simulink model "D24P414_1_model02"  (R2021a)
settings: Solver=VariableStepAuto  StartTime=0.0  StopTime=7  FixedStep=1e-6  RelTol=1e-3
values from neighbouring files (symbols this model uses):
  p_ic = climate_p    [D24P414_1_script.m]
  params_fruit = fruit_p    [D24P414_1_script.m]
  t0_shift = days(t0-t0_12_00)    [D24P414_1_script.m]
  x0_fruit = fruit_ic    [D24P414_1_script.m]
  x0_ic = climate_ic    [D24P414_1_script.m]
libraries: HORTISIM x14
(part 2 of 2)

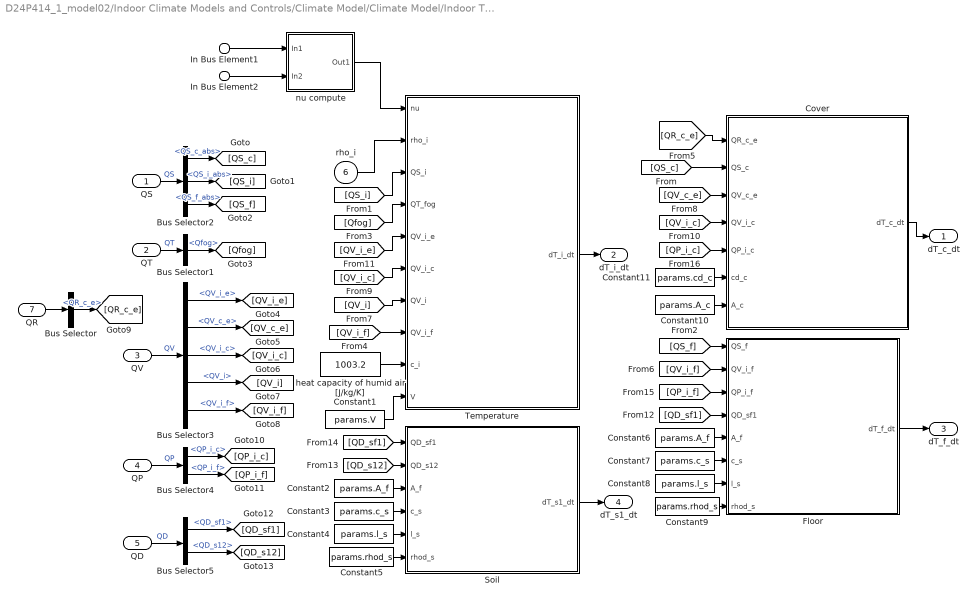
== system D24P414_1_model02/Indoor Climate Models and Controls/Climate Model/Climate Model/Indoor Temperature Model/Heat Balance ==
  QS : Inport
  QT : Inport  Port=2
  QV : Inport  Port=3
  QP : Inport  Port=4
  QD : Inport  Port=5
  rho_i : Inport  Port=6
  QR : Inport  Port=7
  In Bus Element1 : Inport  Port=8  PortName=screen  Element=beta
  In Bus Element2 : Inport  Port=8  PortName=screen  Element=value
  " Cover" : MATLAB Function  TreatAsAtomicUnit=on
  " Floor" : MATLAB Function  TreatAsAtomicUnit=on
  " Soil" : MATLAB Function  TreatAsAtomicUnit=on
  " Temperature" : MATLAB Function  TreatAsAtomicUnit=on
  Bus Selector : BusSelector  OutputSignals=QR_c_e
  Bus Selector1 : BusSelector  OutputSignals=Qfog
  Bus Selector2 : BusSelector  OutputSignals=QS_c_abs,QS_i_abs,QS_f_abs
  Bus Selector3 : BusSelector  OutputSignals=QV_i_e,QV_c_e,QV_i_c,QV_i,QV_i_f
  Bus Selector4 : BusSelector  OutputSignals=QP_i_c,QP_i_f
  Bus Selector5 : BusSelector  OutputSignals=QD_sf1,QD_s12
  Constant1 : Constant  Value=params.V
  Constant10 : Constant  Value=params.A_c
  Constant11 : Constant  Value=params.cd_c
  Constant2 : Constant  Value=params.A_f
  Constant3 : Constant  Value=params.c_s
  Constant4 : Constant  Value=params.l_s
  Constant5 : Constant  Value=params.rhod_s
  Constant6 : Constant  Value=params.A_f
  Constant7 : Constant  Value=params.c_s
  Constant8 : Constant  Value=params.l_s
  Constant9 : Constant  Value=params.rhod_s
  "heat capacity of humid air [J/kg/K] " : Constant  Value=1003.2
  nu compute : Subsystem
  dT_c_dt : Outport
  dT_i_dt : Outport  Port=2
  dT_f_dt : Outport  Port=3
  dT_s1_dt : Outport  Port=4
  wires:
  [QR_c_e] -> " Cover"/1(QR_c_e)
  Bus Selector/1 -> [QR_c_e]  "<QR_c_e>"
  QR/1 -> Bus Selector/1
  Constant11/1 -> " Cover"/6(cd_c)
  Constant10/1 -> " Cover"/7(A_c)
  Constant9/1 -> " Floor"/8(rhod_s)
  Constant8/1 -> " Floor"/7(l_s)
  Constant7/1 -> " Floor"/6(c_s)
  Constant6/1 -> " Floor"/5(A_f)
  Constant5/1 -> " Soil"/6(rhod_s)
  Constant4/1 -> " Soil"/5(l_s)
  Constant3/1 -> " Soil"/4(c_s)
  Constant2/1 -> " Soil"/3(A_f)
  Constant1/1 -> " Temperature"/10(V)
  "heat capacity of humid air [J/kg/K] "/1 -> " Temperature"/9(c_i)
  [QP_i_c] -> " Cover"/5(QP_i_c)
  [QP_i_f] -> " Floor"/3(QP_i_f)
  [QD_sf1] -> " Soil"/1(QD_sf1)
  [QD_s12] -> " Soil"/2(QD_s12)
  [QD_sf1] -> " Floor"/4(QD_sf1)
  Bus Selector5/2 -> [QD_s12]  "<QD_s12>"
  Bus Selector5/1 -> [QD_sf1]  "<QD_sf1>"
  Bus Selector4/2 -> [QP_i_f]  "<QP_i_f>"
  Bus Selector4/1 -> [QP_i_c]  "<QP_i_c>"
  [QV_i_e] -> " Temperature"/5(QV_i_e)
  [QV_i_c] -> " Cover"/4(QV_i_c)
  [QV_i_c] -> " Temperature"/6(QV_i_c)
  [QV_c_e] -> " Cover"/3(QV_c_e)
  [QV_i] -> " Temperature"/7(QV_i)
  [QV_i_f] -> " Floor"/2(QV_i_f)
  [QV_i_f] -> " Temperature"/8(QV_i_f)
  Bus Selector3/2 -> [QV_c_e]  "<QV_c_e>"
  Bus Selector3/3 -> [QV_i_c]  "<QV_i_c>"
  Bus Selector3/4 -> [QV_i]  "<QV_i>"
  Bus Selector3/5 -> [QV_i_f]  "<QV_i_f>"
  Bus Selector3/1 -> [QV_i_e]  "<QV_i_e>"
  [Qfog] -> " Temperature"/4(QT_fog)
  Bus Selector1/1 -> [Qfog]  "<Qfog>"
  [QS_f] -> " Floor"/1(QS_f)
  [QS_i] -> " Temperature"/3(QS_i)
  [QS_c] -> " Cover"/2(QS_c)
  Bus Selector2/3 -> [QS_f]  "<QS_f_abs>"
  Bus Selector2/2 -> [QS_i]  "<QS_i_abs>"
  Bus Selector2/1 -> [QS_c]  "<QS_c_abs>"
  " Cover"/1(dT_c_dt) -> dT_c_dt/1
  QV/1 -> Bus Selector3/1  "QV"
  rho_i/1 -> " Temperature"/2(rho_i)
  QP/1 -> Bus Selector4/1  "QP"
  QS/1 -> Bus Selector2/1  "QS"
  QT/1 -> Bus Selector1/1  "QT"
  " Temperature"/1(dT_i_dt) -> dT_i_dt/1
  QD/1 -> Bus Selector5/1  "QD"
  " Soil"/1(dT_s1_dt) -> dT_s1_dt/1
  " Floor"/1(dT_f_dt) -> dT_f_dt/1
  In Bus Element1/1 -> nu compute/1(In1)
  In Bus Element2/1 -> nu compute/2(In2)
  nu compute/1(Out1) -> " Temperature"/1(nu)

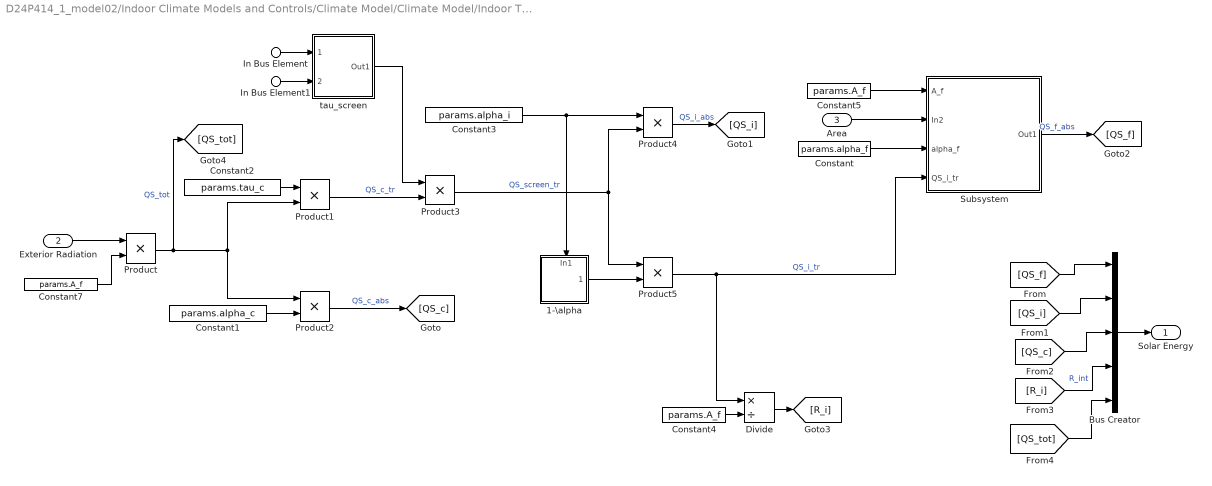
== system D24P414_1_model02/Indoor Climate Models and Controls/Climate Model/Climate Model/Indoor Temperature Model/Radiation Model ==
  In Bus Element : Inport  PortName=screen  Element=gamma_max
  In Bus Element1 : Inport  PortName=screen  Element=value
  Exterior Radiation : Inport  Port=2
  Area : Inport  Port=3
  1-\alpha : Subsystem
      settings: PortSchema="{\"entries\":[{\"content\":{\"sides\":[{\"content\":{\"connectorIds\":[]},\"type\":\"ConnectorPlacement.EquallySpacedRectSide\",\"uuid\":\"bf116baa-1c91-42ba-b5ce-6949a5122443\"},{\"content\":{\"connectorIds\":[\"Out1\"],\"side\":\"RIGHT\"},\"type\":\"ConnectorPlacement.EquallySpacedRectSide\",\"uuid\":\"479b2a41-aae8-4d0f-95ce-40d0c52850dd\"},{\"content\":{\"connectorIds\":[\"In1\"],\"side\":\"TOP\"},\"type\":\"ConnectorPlacement.EquallySpacedRectSide\",\"uuid\":\"d0364cd7-422a-4274-8084-cbaa88b34f4b\"}]},\"type\":\"ConnectorPlacement.EquallySpacedConnector\",\"uuid\":\"3d8ba820-72ed-4082-b0d9-d7ce7398093f\"}],\"packageUris\":[\"http://schema.mathworks.com/mf0/Connector/R2020b\"],\"version\":\"1.0\"}"
  Bus Creator : BusCreator  Inputs=5
  Constant : Constant  Value=params.alpha_f
  Constant1 : Constant  Value=params.alpha_c
  Constant2 : Constant  Value=params.tau_c
  Constant3 : Constant  Value=params.alpha_i
  Constant4 : Constant  Value=params.A_f
  Constant5 : Constant  Value=params.A_f
  Constant7 : Constant  Value=params.A_f
  Divide : Product  Inputs=*/
  Product{,1..5} (6 alike) : Product
  Subsystem : Subsystem
  tau_screen : Subsystem
  "Solar Energy  " : Outport
  wires:
  Divide/1 -> [R_i]
  Constant4/1 -> Divide/2
  Subsystem/1(Out1) -> [QS_f]  "QS_f_abs"
  Product5/1 -> Divide/1, Subsystem/4(QS_i_tr)  "QS_i_tr"
  Constant/1 -> Subsystem/3(alpha_f)
  Area/1 -> Subsystem/2(In2)
  Constant5/1 -> Subsystem/1(A_f)
  Product4/1 -> [QS_i]  "QS_i_abs"
  1-\alpha/1(Out1) -> Product5/2
  Constant3/1 -> 1-\alpha/1(In1), Product4/1
  Product3/1 -> Product5/1, Product4/2  "QS_screen_tr"
  tau_screen/1(Out1) -> Product3/1
  Product2/1 -> [QS_c]  "QS_c_abs"
  Product1/1 -> Product3/2  "QS_c_tr"
  Constant1/1 -> Product2/2
  Constant2/1 -> Product1/1
  Product/1 -> [QS_tot], Product1/2, Product2/1  "QS_tot"
  Constant7/1 -> Product/2
  Exterior Radiation/1 -> Product/1
  [R_i] -> Bus Creator/4  "R_int"
  [QS_c] -> Bus Creator/3
  Bus Creator/1 -> "Solar Energy  "/1
  [QS_f] -> Bus Creator/1
  [QS_i] -> Bus Creator/2
  [QS_tot] -> Bus Creator/5
  In Bus Element1/1 -> tau_screen/2(screen)
  In Bus Element/1 -> tau_screen/1(gamma)

== system D24P414_1_model02/Indoor Climate Models and Controls/Climate Model/Climate Model/Indoor Temperature Model/Subsystem ==
  Tc : Inport
  Te : Inport  Port=2
  " Stefan-Boltzmann constant [W/m^2/K^4] " : Constant  Value=5.67e-8
  Bus Creator : BusCreator  Inputs=1
  Constant : Constant  Value=4
  Constant1 : Constant  Value=4
  Constant2 : Constant  Value=params.A_c
  Minus : Sum  Inputs=+-
  Product : Product  Inputs=4
  Square : Math  Operator=pow  SaturateOnIntegerOverflow=on
  Square1 : Math  Operator=pow  SaturateOnIntegerOverflow=on
  k : Constant  Value=0.985
  QR : Outport
  wires:
  Bus Creator/1 -> QR/1
  Product/1 -> Bus Creator/1  "QR_c_e"
  Constant1/1 -> Square1/2
  " Stefan-Boltzmann constant [W/m^2/K^4] "/1 -> Product/4
  k/1 -> Product/3
  Minus/1 -> Product/1
  Constant2/1 -> Product/2
  Square1/1 -> Minus/2
  Square/1 -> Minus/1
  Te/1 -> Square1/1
  Constant/1 -> Square/2
  Tc/1 -> Square/1

== system D24P414_1_model02/Indoor Climate Models and Controls/Set Point Controler/Heater SetPoints/Subsystem1/Every Day ==
  T_min : Inport
  T_max : Inport  Port=2
  Te : Inport  Port=3
  Action Port : ActionPort  ActionPortLabel=if(u1 == 1)
  Clock : Clock
  Heater Setpoints Calculator : Subsystem
  Subsystem : Subsystem
  T_start : Outport
  T_stop : Outport  Port=2
  wires:
  Heater Setpoints Calculator/2(T_stop) -> T_stop/1  "T_stop"
  T_max/1 -> Heater Setpoints Calculator/2(T_max)
  Heater Setpoints Calculator/1(T_start) -> T_start/1  "T_start"
  T_min/1 -> Heater Setpoints Calculator/1(T_min)
  Subsystem/1(DayChange) -> Heater Setpoints Calculator/Trigger
  Clock/1 -> Heater Setpoints Calculator/3(t)
  Te/1 -> Heater Setpoints Calculator/4(Te)

== system D24P414_1_model02/Indoor Climate Models and Controls/Set Point Controler/Heater SetPoints/Subsystem1/Every Day1 ==
  T_min : Inport
  T_max : Inport  Port=2
  Action Port : ActionPort  ActionPortLabel=elseif(u1==4)
  T_start : Outport
  T_stop : Outport  Port=2
  wires:
  T_min/1 -> T_start/1
  T_max/1 -> T_stop/1

== system D24P414_1_model02/Indoor Climate Models and Controls/Set Point Controler/Heater SetPoints/Subsystem1/Real Time ==
  T_min : Inport
  T_max : Inport  Port=2
  <Temp> : Inport  Port=3
  Action Port : ActionPort  ActionPortLabel=elseif(u1 == 2)
  Constant : Constant  Value=0.5
  Constant1 : Constant  Value=2
  Gain : Gain  Gain=3.5
  Minus : Sum  Inputs=+-
  Square : Math  Operator=pow  SignedPower=on  SaturateOnIntegerOverflow=on
  Sum : Sum  Inputs=|++
  Sum1 : Sum  Inputs=|+++
  T_start : Outport
  T_stop : Outport  Port=2
  wires:
  Sum1/1 -> T_stop/1  "T_stop"
  Sum/1 -> T_start/1  "T_start"
  Gain/1 -> Sum1/2, Sum/2
  T_max/1 -> Sum1/1
  T_min/1 -> Minus/1, Sum/1
  <Temp>/1 -> Minus/2
  Minus/1 -> Square/1
  Square/1 -> Gain/1
  Constant/1 -> Square/2
  Constant1/1 -> Sum1/3

== system D24P414_1_model02/Indoor Climate Models and Controls/Set Point Controler/Heater SetPoints/Subsystem1/Real Time1 ==
  Action Port : ActionPort  ActionPortLabel=elseif(u1 == 3)
  Constant : Constant  Value=20 + 273.15
  Constant1 : Constant  Value=10+273.15
  T_start : Outport
  T_stop : Outport  Port=2
  wires:
  Constant1/1 -> T_start/1  "T_start"
  Constant/1 -> T_stop/1

== system D24P414_1_model02/Indoor Climate Models and Controls/Climate Model/Climate Model/Gases Exchange/Carbon Dynamics/Carbon Exchange Indoor-Outdoor ==
  R_a : Inport
  C_c : Inport  Port=2
  C_ce : Inport  Port=3
  Minus : Sum  Inputs=+-
  Product : Product
  MC_i_e : Outport
  wires:
  Product/1 -> MC_i_e/1
  R_a/1 -> Product/1
  Minus/1 -> Product/2
  C_ce/1 -> Minus/2
  C_c/1 -> Minus/1

== system D24P414_1_model02/Indoor Climate Models and Controls/Climate Model/Climate Model/Gases Exchange/Carbon Dynamics/External CO2 Concentration ==
  T_e : Inport
  Divide : Product  Inputs=**//
  Gain : Gain  Gain=4e-4
  M_c : Constant  Value=0.0440
  R : Constant  Value=8.3140
  atm : Constant  Value=101300
  C_ce : Outport
  wires:
  Gain/1 -> C_ce/1
  Divide/1 -> Gain/1
  T_e/1 -> Divide/4
  M_c/1 -> Divide/2
  R/1 -> Divide/3
  atm/1 -> Divide/1

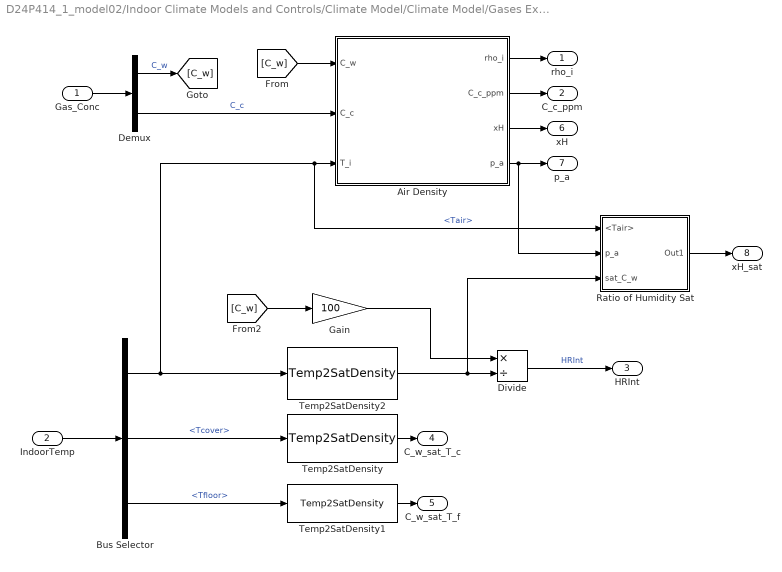
== system D24P414_1_model02/Indoor Climate Models and Controls/Climate Model/Climate Model/Gases Exchange/Compute Mid Variables/Subsystem ==
  Gas_Conc : Inport
  IndoorTemp : Inport  Port=2
  Air Density : MATLAB Function  TreatAsAtomicUnit=on
  Bus Selector : BusSelector  OutputSignals=Tair,Tcover,Tfloor
  Demux : Demux  Outputs=2
  Divide : Product  Inputs=*/
  Gain : Gain  Gain=100
  Ratio of Humidity Sat : Subsystem
  Temp2SatDensity : HORTISIM/Other  Functions/Temp2SatDensity  SystemSampleTime=-1  VariantActivationTime=update diagram  Latency=0  AutoFrameSizeCalculation=off
      settings: SourceProductName=Horti Simulator
  Temp2SatDensity1 : HORTISIM/Other  Functions/Temp2SatDensity  SystemSampleTime=-1  VariantActivationTime=update diagram  Latency=0  AutoFrameSizeCalculation=off
      settings: SourceProductName=Horti Simulator
  Temp2SatDensity2 : HORTISIM/Other  Functions/Temp2SatDensity  SystemSampleTime=-1  VariantActivationTime=update diagram  Latency=0  AutoFrameSizeCalculation=off
      settings: SourceProductName=Horti Simulator
  rho_i : Outport
  C_c_ppm : Outport  Port=2
  HRInt : Outport  Port=3
  C_w_sat_T_c : Outport  Port=4
  C_w_sat_T_f : Outport  Port=5
  xH : Outport  Port=6
  p_a : Outport  Port=7
  xH_sat : Outport  Port=8
  wires:
  Ratio of Humidity Sat/1(Out1) -> xH_sat/1
  Divide/1 -> HRInt/1  "HRInt"
  [C_w] -> Gain/1
  Gain/1 -> Divide/1
  Temp2SatDensity2/1 -> Divide/2, Ratio of Humidity Sat/3(sat_C_w)
  Air Density/4(p_a) -> p_a/1, Ratio of Humidity Sat/2(p_a)
  Air Density/3(xH) -> xH/1
  [C_w] -> Air Density/1(C_w)
  Air Density/2(C_c_ppm) -> C_c_ppm/1
  Air Density/1(rho_i) -> rho_i/1
  Demux/2 -> Air Density/2(C_c)  "C_c"
  Demux/1 -> [C_w]  "C_w"
  Temp2SatDensity1/1 -> C_w_sat_T_f/1
  Temp2SatDensity/1 -> C_w_sat_T_c/1
  Bus Selector/3 -> Temp2SatDensity1/1  "<Tfloor>"
  Bus Selector/2 -> Temp2SatDensity/1  "<Tcover>"
  Gas_Conc/1 -> Demux/1
  Bus Selector/1 -> Temp2SatDensity2/1, Air Density/3(T_i), Ratio of Humidity Sat/1(<Tair>)  "<Tair>"
  IndoorTemp/1 -> Bus Selector/1

== system D24P414_1_model02/Indoor Climate Models and Controls/Climate Model/Climate Model/Gases Exchange/Water Dynamics/Subsystem ==
  <Temperature> : Inport
  <Exterior Humidity> : Inport  Port=2
  Gain : Gain  Gain=1/100
  Product : Product
  Temp2SatDensity : HORTISIM/Other  Functions/Temp2SatDensity  SystemSampleTime=-1  VariantActivationTime=update diagram  Latency=0  AutoFrameSizeCalculation=off
      settings: SourceProductName=Horti Simulator
  C_w_Te : Outport
  wires:
  Gain/1 -> Product/2
  Temp2SatDensity/1 -> Product/1  "C_w_sat_Te"
  <Exterior Humidity>/1 -> Gain/1
  <Temperature>/1 -> Temp2SatDensity/1
  Product/1 -> C_w_Te/1  "C_w_Te"

== system D24P414_1_model02/Indoor Climate Models and Controls/Climate Model/Climate Model/Gases Exchange/Water Dynamics/Vapor Mass Balance ==
  <QT_v_i> : Inport
  <Qfog> : Inport  Port=2
  MW_i_e : Inport  Port=3
  <QP_i_c> : Inport  Port=4
  <QP_i_f> : Inport  Port=5
  Constant1 : Constant  Value=params.V
  Divide : Product  Inputs=*/
  Divide1 : Product  Inputs=*/
  Minus : Sum  Inputs=+-
  Product : Product
  Scope : Scope
  Scope1 : Scope
  Sum : Sum  Inputs=|+--+
  latent heat of condensation of water [J/kg] : Constant  Value=2437000
  dC_w_dt : Outport
  wires:
  Divide1/1 -> Scope/1
  Minus/1 -> dC_w_dt/1
  MW_i_e/1 -> Minus/2
  Divide/1 -> Minus/1
  Product/1 -> Divide/2, Divide1/2
  Sum/1 -> Divide/1
  <Qfog>/1 -> Sum/4
  <QP_i_f>/1 -> Sum/3
  <QP_i_c>/1 -> Sum/2, Scope1/1
  <QT_v_i>/1 -> Sum/1, Divide1/1
  Constant1/1 -> Product/2
  latent heat of condensation of water [J/kg]/1 -> Product/1

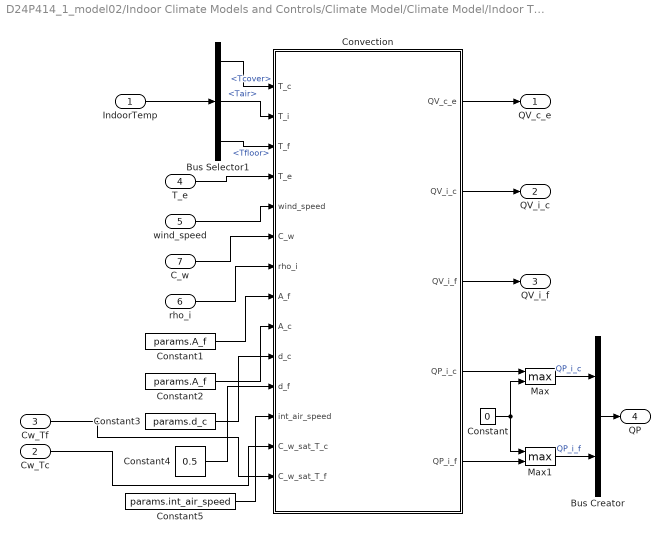
== system D24P414_1_model02/Indoor Climate Models and Controls/Climate Model/Climate Model/Indoor Temperature Model/Convection/Convection ==
  IndoorTemp : Inport
  Cw_Tc : Inport  Port=2
  Cw_Tf : Inport  Port=3
  T_e : Inport  Port=4
  wind_speed : Inport  Port=5
  rho_i : Inport  Port=6
  C_w : Inport  Port=7
  Bus Creator : BusCreator  Inputs=2
  Bus Selector1 : BusSelector  OutputSignals=Tcover,Tair,Tfloor
  Constant : Constant  Value=0
  Constant1 : Constant  Value=params.A_f
  Constant2 : Constant  Value=params.A_f
  Constant3 : Constant  Value=params.d_c
  Constant4 : Constant  Value=0.5
  Constant5 : Constant  Value=params.int_air_speed
  Convection : MATLAB Function  TreatAsAtomicUnit=on
  Max : MinMax  Function=max  Inputs=2
  Max1 : MinMax  Function=max  Inputs=2
  QV_c_e : Outport
  QV_i_c : Outport  Port=2
  QV_i_f : Outport  Port=3
  QP : Outport  Port=4
  wires:
  Cw_Tc/1 -> Convection/13(C_w_sat_T_c)
  Cw_Tf/1 -> Convection/14(C_w_sat_T_f)
  Constant5/1 -> Convection/12(int_air_speed)
  Constant4/1 -> Convection/11(d_f)
  Constant3/1 -> Convection/10(d_c)
  Constant2/1 -> Convection/9(A_c)
  Constant1/1 -> Convection/8(A_f)
  wind_speed/1 -> Convection/5(wind_speed)
  T_e/1 -> Convection/4(T_e)
  Bus Selector1/3 -> Convection/3(T_f)  "<Tfloor>"
  Bus Selector1/2 -> Convection/2(T_i)  "<Tair>"
  Bus Selector1/1 -> Convection/1(T_c)  "<Tcover>"
  IndoorTemp/1 -> Bus Selector1/1
  Max/1 -> Bus Creator/1  "QP_i_c"
  Max1/1 -> Bus Creator/2  "QP_i_f"
  Convection/4(QP_i_c) -> Max/1
  Convection/5(QP_i_f) -> Max1/2
  Constant/1 -> Max/2, Max1/1
  rho_i/1 -> Convection/7(rho_i)
  C_w/1 -> Convection/6(C_w)
  Bus Creator/1 -> QP/1
  Convection/3(QV_i_f) -> QV_i_f/1
  Convection/2(QV_i_c) -> QV_i_c/1
  Convection/1(QV_c_e) -> QV_c_e/1

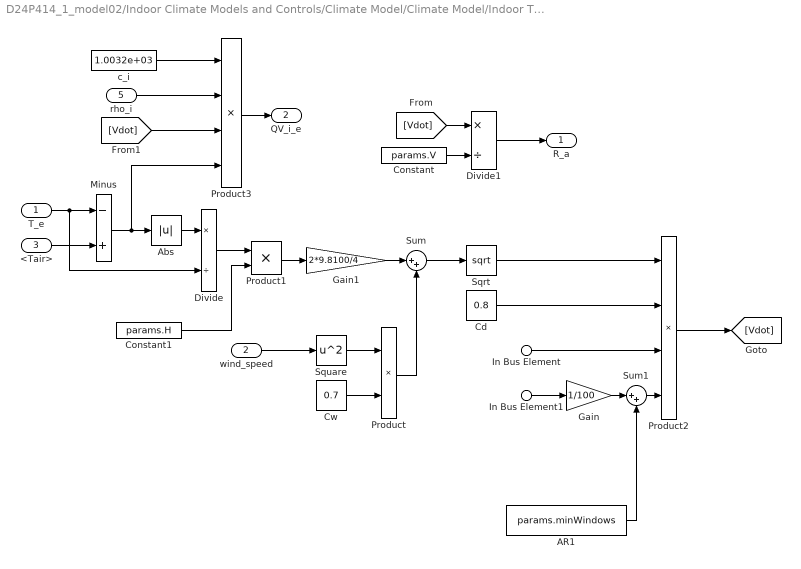
== system D24P414_1_model02/Indoor Climate Models and Controls/Climate Model/Climate Model/Indoor Temperature Model/Convection/Subsystem ==
  T_e : Inport
  wind_speed : Inport  Port=2
  <Tair> : Inport  Port=3
  In Bus Element1 : Inport  Port=4  PortName=Windows  Element=value
  In Bus Element : Inport  Port=4  PortName=Windows  Element=AR
  rho_i : Inport  Port=5
  AR1 : Constant  Value=params.minWindows  VectorParams1D=off
  Abs : Abs  ZeroCross=off
  Cd : Constant  Value=0.8  VectorParams1D=off
  Constant : Constant  Value=params.V
  Constant1 : Constant  Value=params.H
  Cw : Constant  Value=0.7  VectorParams1D=off
  Divide : Product  Inputs=*/
  Divide1 : Product  Inputs=*/
  Gain : Gain  Gain=1/100
  Gain1 : Gain  Gain=2*9.8100/4
  Minus : Sum  Inputs=-+
  Product : Product
  Product1 : Product
  Product2 : Product  Inputs=4
  Product3 : Product  Inputs=4
  Sqrt : Sqrt  SaturateOnIntegerOverflow=on
  Square : Math  Operator=square  SaturateOnIntegerOverflow=on
  Sum : Sum  Inputs=|++
  Sum1 : Sum  Inputs=|++
  c_i : Constant  Value=1.0032e+03  VectorParams1D=off
  R_a : Outport
  QV_i_e : Outport  Port=2
  wires:
  AR1/1 -> Sum1/2
  Sum1/1 -> Product2/4
  Gain/1 -> Sum1/1
  Product3/1 -> QV_i_e/1
  c_i/1 -> Product3/1
  rho_i/1 -> Product3/2
  [Vdot] -> Product3/3
  Divide1/1 -> R_a/1
  Constant/1 -> Divide1/2
  [Vdot] -> Divide1/1
  Product2/1 -> [Vdot]
  Cd/1 -> Product2/2
  Sqrt/1 -> Product2/1
  Sum/1 -> Sqrt/1
  Gain1/1 -> Sum/1
  Product1/1 -> Gain1/1
  Divide/1 -> Product1/1
  Constant1/1 -> Product1/2
  Abs/1 -> Divide/1
  Minus/1 -> Abs/1, Product3/4
  <Tair>/1 -> Minus/2
  T_e/1 -> Divide/2, Minus/1
  Product/1 -> Sum/2
  Cw/1 -> Product/2
  Square/1 -> Product/1
  wind_speed/1 -> Square/1
  In Bus Element1/1 -> Gain/1
  In Bus Element/1 -> Product2/3

== system D24P414_1_model02/Indoor Climate Models and Controls/Climate Model/Climate Model/Indoor Temperature Model/Heat Balance/nu compute ==
  In1 : Inport
  In2 : Inport  Port=2
  Constant : Constant
  Gain : Gain  Gain=1/100
  Product : Product
  Scope : Scope
  Sum : Sum  Inputs=|++
  Out1 : Outport
  wires:
  Sum/1 -> Scope/1, Out1/1
  In1/1 -> Product/1
  Constant/1 -> Sum/2
  In2/1 -> Gain/1
  Product/1 -> Sum/1
  Gain/1 -> Product/2

== system D24P414_1_model02/Indoor Climate Models and Controls/Climate Model/Climate Model/Indoor Temperature Model/Radiation Model/1-\alpha ==
  In1 : Inport
  Constant6 : Constant
  Minus : Sum  Inputs=+-
  Out1 : Outport
  wires:
  Constant6/1 -> Minus/1
  In1/1 -> Minus/2
  Minus/1 -> Out1/1

== system D24P414_1_model02/Indoor Climate Models and Controls/Climate Model/Climate Model/Indoor Temperature Model/Radiation Model/Subsystem ==
  A_f : Inport
  In2 : Inport  Port=2
  alpha_f : Inport  Port=3
  QS_i_tr : Inport  Port=4
  Divide : Product  Inputs=*/**
  Minus : Sum  Inputs=+-
  Out1 : Outport
  wires:
  Minus/1 -> Divide/1
  alpha_f/1 -> Divide/3
  In2/1 -> Minus/2
  Divide/1 -> Out1/1
  A_f/1 -> Minus/1, Divide/2
  QS_i_tr/1 -> Divide/4

== system D24P414_1_model02/Indoor Climate Models and Controls/Climate Model/Climate Model/Indoor Temperature Model/Radiation Model/tau_screen ==
  gamma : Inport
  screen : Inport  Port=2
  Constant3 : Constant
  Divide : Product  Inputs=**
  Gain : Gain  Gain=1/100
  Minus : Sum  Inputs=+-
  Out1 : Outport
  wires:
  Constant3/1 -> Minus/1
  screen/1 -> Divide/2
  Minus/1 -> Out1/1
  Gain/1 -> Minus/2
  Divide/1 -> Gain/1
  gamma/1 -> Divide/1

== system D24P414_1_model02/Indoor Climate Models and Controls/Set Point Controler/Heater SetPoints/Subsystem1/Every Day/Heater Setpoints Calculator ==
  T_min : Inport
  T_max : Inport  Port=2
  t : Inport  Port=3
  Te : Inport  Port=4
  Trigger : TriggerPort  TriggerType=either  VariantControl=(inherit)
  Gain : Gain  Gain=2
  MATLAB Function : MATLAB Function  Commented=through  TreatAsAtomicUnit=on
  Minus : Sum  Inputs=+-
  Sum : Sum  Inputs=|++
  Sum1 : Sum  Inputs=|++
  T_start : Outport
  T_stop : Outport  Port=2
  wires:
  T_min/1 -> Minus/1, Sum/1
  Sum/1 -> T_start/1
  Sum1/1 -> T_stop/1
  T_max/1 -> Sum1/1
  Gain/1 -> Sum1/2, Sum/2
  Minus/1 -> Gain/1
  t/1 -> MATLAB Function/1(u)
  Te/1 -> Minus/2

== system D24P414_1_model02/Indoor Climate Models and Controls/Set Point Controler/Heater SetPoints/Subsystem1/Every Day/Subsystem ==
  Clock : Clock
  If : If  IfExpression=u1 == 0
  If Action Subsystem : Subsystem  TreatAsAtomicUnit=on
  If Action Subsystem1 : Subsystem  TreatAsAtomicUnit=on
  Merge : Merge
  DayChange : Outport
  wires:
  Merge/1 -> DayChange/1
  Clock/1 -> If Action Subsystem1/1(In1), If/1
  If/1 -> If Action Subsystem/Action
  If/2 -> If Action Subsystem1/Action
  If Action Subsystem/1(Out1) -> Merge/1
  If Action Subsystem1/1(Out1) -> Merge/2

== system D24P414_1_model02/Indoor Climate Models and Controls/Climate Model/Climate Model/Gases Exchange/Compute Mid Variables/Subsystem/Ratio of Humidity Sat ==
  <Tair> : Inport
  p_a : Inport  Port=2
  sat_C_w : Inport  Port=3
  " molar mass of water [kg/mol]" : Constant  Value=0.0180
  Divide1 : Product  Inputs=*/
  Divide2 : Product  Inputs=*/
  Gain1 : Gain  Gain=0.62198
  Minus : Sum  Inputs=+-
  Product : Product  Inputs=3
  gas constant [J/mol/K] : Constant  Value=8.3140
  Out1 : Outport
  wires:
  Divide2/1 -> Gain1/1
  Divide1/1 -> Minus/2, Divide2/1  "p_w^*"
  gas constant [J/mol/K]/1 -> Product/2
  " molar mass of water [kg/mol]"/1 -> Divide1/2
  Product/1 -> Divide1/1
  <Tair>/1 -> Product/1
  sat_C_w/1 -> Product/3
  Gain1/1 -> Out1/1
  Minus/1 -> Divide2/2
  p_a/1 -> Minus/1

== system D24P414_1_model02/Indoor Climate Models and Controls/Set Point Controler/Heater SetPoints/Subsystem1/Every Day/Subsystem/If Action Subsystem ==
  Action Port : ActionPort  ActionPortLabel=if(u1 == 0)
  Constant : Constant  Value=0
  Out1 : Outport
  wires:
  Constant/1 -> Out1/1

== system D24P414_1_model02/Indoor Climate Models and Controls/Set Point Controler/Heater SetPoints/Subsystem1/Every Day/Subsystem/If Action Subsystem1 ==
  In1 : Inport
  Action Port : ActionPort  ActionPortLabel=else
  Constant1 : Constant  Value=t0_shift
  Gain : Gain  Gain=pi
  Sin : Trigonometry
  Sum : Sum  Inputs=|++
  Out1 : Outport
  wires:
  Constant1/1 -> Sum/2
  Gain/1 -> Sin/1
  Sum/1 -> Gain/1
  In1/1 -> Sum/1
  Sin/1 -> Out1/1

== matlab function D24P414_1_model02/Indoor Climate Models and Controls/Climate Model/Climate Model/Indoor Temperature Model/Conduction/Conduction ==
  data: T_f input; T_s1 input; QD_sf1 output; QD_s12 output; A_f input; lam_s input; l_s input; T_ss input
function [QD_sf1,QD_s12] = fcn(T_f,T_s1,A_f,lam_s,l_s,T_ss)

%
%%
% GEOMETRY
% ========
% A_f = p.A_f; % greenhouse floor area [m^2]
% 
% % FLOOR 
% % =====================
% lam_s= p.lam_s; %thermal conductivity of soil layers [W/mK] Concrete, Soil, Clay
% l_s  = p.l_s; %thickness of soil layers [m]
% 
% T_ss = p.T_ss; %deep soil temperature [K]

%%      Conduction
% Floor layers 
% 
QD_sf1 = A_f*lam_s(1)/l_s(1).*(T_f - T_s1); 
QD_s12 = A_f*lam_s(2)/l_s(2).*(T_s1 - T_ss);

== matlab function D24P414_1_model02/Indoor Climate Models and Controls/Climate Model/Climate Model/Indoor Temperature Model/Convection/Convection/Convection ==
  data: QV_c_e output; QV_i_c output; QV_i_f output; T_c input; T_i input; T_f input; T_e input; wind_speed input; QP_i_c output; QP_i_f output; C_w input; rho_i input; A_f input; A_c input; d_c input; d_f input; int_air_speed input; C_w_sat_T_c input; C_w_sat_T_f input
function [QV_c_e,QV_i_c,QV_i_f,QP_i_c,QP_i_f] = fcn( T_c,T_i,T_f,T_e,wind_speed,C_w,rho_i,A_f,A_c,d_c,d_f,int_air_speed,C_w_sat_T_c,C_w_sat_T_f)

% CONSTANTS
% =========
g = 9.8100; % acceleration due to gravity [m/s^2]
lambda = 0.0250; % thermal conductivity of air [W/m/K]

Le = 0.8190; % Lewis number [-] 
nu =  1.5100e-05; % kinematic viscosity [m^2/s]

%%
c_i = 1.0032e+03;
H_fg = 2437000;

%%

if wind_speed<0
    wind_speed = 0;
end
%%      Convection

% The Grashof and Reynolds numbers are calculated, and then the Nusselt
% number calculated as the larger of the 'free' Nusselt number, based on
% the Grashof number, and the 'forced' Nusselt number, based on the
% Reynolds number. The heat transferred per unit time is then calculated
% based on this. The first subscript is where heat is transferred from, and
% the second subscript where heat is transferred to.

% Cover to external air
Gr = g*d_c^3/(T_e*nu^2)*abs(T_c - T_e);
Re = wind_speed*d_c/nu;
Nu = lamorturb(Gr, Re);
QV_c_e = 4*A_c.*Nu*lambda.*(T_c - T_e)/d_c;

% Internal air to cover
Gr = g*d_c^3./(T_i*nu^2).*abs(T_i - T_c);
Re = int_air_speed*d_c/nu;  
[Nu, Sh] = lamorturb(Gr, Re, Le);
QV_i_c = 4*A_c.*Nu*lambda.*(T_i - T_c)/d_c;
QP_i_c = 4*A_c*H_fg./(rho_i*c_i).*Sh/Le*lambda/d_c.*(C_w - C_w_sat_T_c);
%QP_i_c = max(QP_i_c,0); % assumed no evaporation from the cover, only condensation

%Internal air to floor
Gr = g*d_f^3./(T_i*nu^2).*abs(T_i - T_f); 
Re = int_air_speed*d_f/nu;
[Nu, Sh] = lamorturb(Gr, Re, Le);
QV_i_f = A_f.*Nu*lambda.*(T_i - T_f)/d_f;
QP_i_f = A_f*H_fg./(rho_i*c_i).*Sh/Le*lambda/d_f.*(C_w - C_w_sat_T_f); 
%QP_i_f = max(QP_i_f,0); % assumed no evaporation from the floor, only condensation

== matlab function D24P414_1_model02/Fruit Partitioning1/MATLAB Function ==
  data: Cfruit input; dCmdt output; Tsum input; Cfruit_mature input; T input; DT output
function [dCmdt,DT] = fcn(Cfruit, Tsum, Cfruit_mature,T)

a = 0.05;

T = T-273.15;
DT = a*max(0,min(1,0.0714*(T-9)));

dCmdt = (Tsum<2600)*DT*(Tsum>1200)*(Cfruit-Cfruit_mature);

== matlab function D24P414_1_model02/Indoor Climate Models and Controls/Set Point Controler/Heater SetPoints/Subsystem1/Every Day/Heater Setpoints Calculator/MATLAB Function ==
  data: u input; y output
function y = fcn(u)

y = MeanTemperaturePred(u);

== matlab function D24P414_1_model02/Indoor Climate Models and Controls/Climate Model/Climate Model/Indoor Temperature Model/Heat Balance/ Soil ==
  data: QD_sf1 input; QD_s12 input; dT_s1_dt output; A_f input; c_s input; l_s input; rhod_s input
function dT_s1_dt  = fcn(QD_sf1,QD_s12,A_f,c_s,l_s,rhod_s)



%% Soil 1
c_Ts1 = 1./(rhod_s(2) * c_s(2) * l_s(2)*A_f);
%
dT_s1_dt = c_Ts1*(QD_sf1 - QD_s12);
%%

== matlab function D24P414_1_model02/Indoor Climate Models and Controls/Climate Model/Climate Model/Indoor Temperature Model/Heat Balance/ Cover ==
  data: QR_c_e input; QS_c input; QV_c_e input; QV_i_c input; QP_i_c input; dT_c_dt output; cd_c input; A_c input
function dT_c_dt = fcn(QR_c_e, QS_c,QV_c_e,QV_i_c,QP_i_c,cd_c,A_c)

%% Cover Temperature
dT_c_dt = 1./(A_c*cd_c).*(+QV_i_c   - QV_c_e  + QS_c + QP_i_c - QR_c_e);

== matlab function D24P414_1_model02/Indoor Climate Models and Controls/Set Point Controler/Triggered Subsystem/MATLAB Function ==
  data: T_min output; T_opt_min output; Tsum input; Rad input; THRad input; T_opt_max output; Tmax output
function [T_min,T_opt_min,T_opt_max,Tmax] = fcn(Tsum, Rad,THRad)


r = OptimalGrowthTemperature(Tsum,Rad,THRad);
r = r + 273.15;

T_min = r(1);
T_opt_min = r(2);
T_opt_max = r(3);
Tmax = r(4);


end
%

function x = OptimalGrowthTemperature(Tsum,Rad,THRad)
    if size(Tsum,2)~=1
       error('Tsum debe ser una columna') 
    end
    x = (Rad> THRad).*OptimalGrowthTemperatureDay(Tsum) + ...
        (Rad<= THRad).*OptimalGrowthTemperatureNight(Tsum);
end


function x = OptimalGrowthTemperatureDay(Tsum)
    if size(Tsum,2)~=1
       error('Tsum debe ser una columna') 
    end
    
        % Tmin Topt_min Topt_max Tmax
    x =   [11      18      25     40  ].*theta(400,Tsum) + ...
          [12      21      24     35  ].*theta(Tsum,400).*theta(1800,Tsum) + ...
          [15      20      25     30  ].*theta(Tsum,1800);  
end

function x = OptimalGrowthTemperatureNight(Tsum)
    if size(Tsum,2)~=1
       error('Tsum debe ser una columna') 
    end
    x = [11 15 18 30 ].*theta(400,Tsum) + ...
        [13 14 14 14].*theta(Tsum,400).*theta(1800,Tsum) + ...
        [10 14 30 35].*theta(Tsum,1800);  
end


function r = theta(x,y)
    eta = 10;
    r = 0.5 + 0.5*tanh(eta*(x-y));
end

== matlab function D24P414_1_model02/Indoor Climate Models and Controls/Climate Model/Climate Model/Indoor Temperature Model/Heat Balance/ Floor ==
  data: QS_f input; QV_i_f input; QP_i_f input; QD_sf1 input; dT_f_dt output; A_f input; c_s input; l_s input; rhod_s input
function dT_f_dt  = fcn(QS_f,QV_i_f,QP_i_f,QD_sf1,A_f,c_s,l_s,rhod_s)



%% Floor
c_Tf =  1./(rhod_s(1) * A_f * c_s(1) * l_s(1));
%
dT_f_dt  =c_Tf*(QV_i_f  + QS_f - QD_sf1 + QP_i_f);

== matlab function D24P414_1_model02/Indoor Climate Models and Controls/Climate Model/Climate Model/Gases Exchange/Compute Mid Variables/Subsystem/Air Density ==
  data: C_w input; C_c input; T_i input; rho_i output; C_c_ppm output; xH output; p_a output
function [rho_i,C_c_ppm,xH,p_a] =   Air(C_w,C_c,T_i)

% CONSTANTS
% =========  
atm = 101300; % standard atmospheric pressure [Pa]
M_a = 0.0290; % molar mass of dry air [kg/mol]                                                                 
R   = 8.3140; % gas constant [J/mol/K]
M_w = 0.0180; % molar mass of water [kg/mol]
M_c = 0.0440; % molar mass of CO2 [kg/mol]


%%
p_w = C_w*R.*T_i/M_w; % Partial pressure of water [Pa]
p_a = (atm - p_w);
rho_i  = (p_a*M_a + p_w*M_w)./(R*T_i); % Density of air [kg/m^3]
C_c_ppm = C_c*R.*T_i/(M_c*atm)*1e6; % CO2 concentration in ppm

xH = 0.62198* p_w /(p_a - p_w);
%%

== matlab function D24P414_1_model02/Indoor Climate Models and Controls/Climate Model/Climate Model/Indoor Temperature Model/Heat Balance/ Temperature ==
  data: nu input; rho_i input; QS_i input; QT_fog input; QV_i_e input; QV_i_c input; QV_i input; QV_i_f input; dT_i_dt output; c_i input; V input
function dT_i_dt  = fcn( nu, rho_i ,QS_i,QT_fog,QV_i_e,QV_i_c,QV_i,QV_i_f,c_i,V)


%% Air Temperature

c_Ti = 1./(nu*V.*rho_i*c_i);

dT_i_dt = c_Ti*(  QV_i - QV_i_f - QV_i_c - QV_i_e + QS_i  - QT_fog); 
%%
